simulink model "PV_panel"  (Simulink 10.0)
settings: Solver=ode45  StartTime=0.0  StopTime=0.2  RelTol=1e-3  EnableMultiTasking=on
undefined symbols (not defined in the file): sigbuilder_block
libraries: fl_lib x5, nesl_utility x5, simulink x3, ee_lib x1
settings Model: Creator=Shivananda  LastModifiedBy=bhisma
settings DataIOCC: LimitDataPoints=on  SignalLoggingSaveFormat=ModelDataLogs
settings OptimizationCC: ExpressionDepthLimit=2147483647
settings DebuggingCC: SolverPrmCheckMsg=warning  FcnCallInpInsideContextMsg=warning  StateNameClashWarn=warning
settings GRTTargetCC: GeneratePreprocessorConditionals=Disable all
settings ConfigComp: CovExternalEMLEnable=off
settings SimscapeCC: SimscapeNormalizeSystem=off

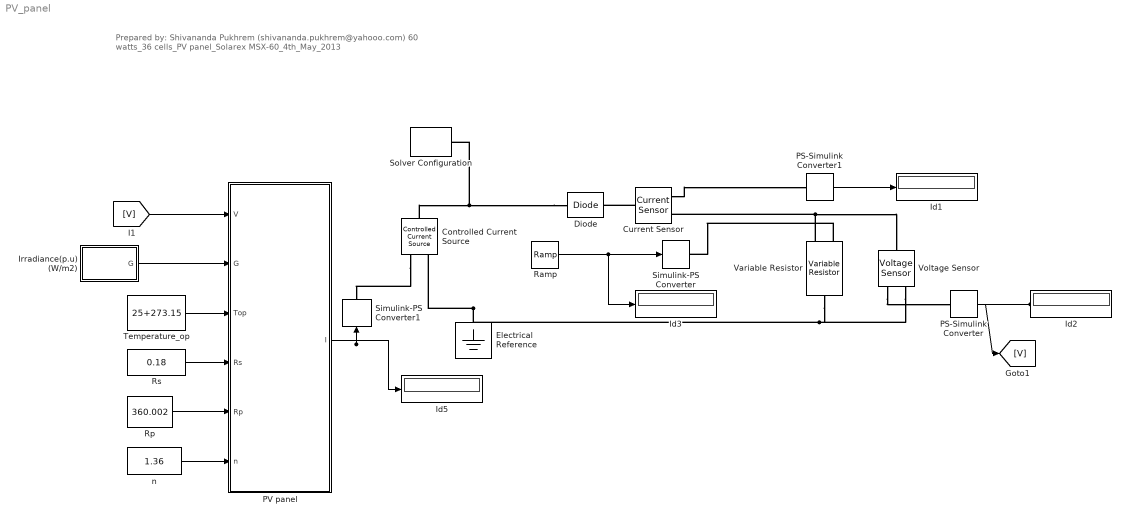
== system PV_panel ==
  note: Prepared by: Shivananda Pukhrem (shivananda.pukhrem@yahooo.com)
      |                          60 watts_36 cells_PV panel_Solarex MSX-60_4th_May_2013
  Controlled Current Source : fl_lib/Electrical/Electrical Sources/Controlled Current Source
  Current Sensor : fl_lib/Electrical/Electrical Sensors/Current Sensor
  Diode : ee_lib/Semiconductors & Converters/Diode  ModelType=ee.enum.diode.modelType.exponential  Vf=0.6 V  Ron=0.3 Ohm  Goff=1e-08 S  prmExp=1  I12="[  0.07 2.2 ] A"  V12="[  15 21 ] V"  IS=1.541765286972375e-008 A  ec=1  I1=0.07 A  V1=0.7 V  RS=0.001 Ohm  Tmeas=25 C  N_series=1  N_parallel=1  Rz=0.3 Ohm  BV=Inf V  C_param=1  CJ=0 pF  CJ0=0 pF  VJ=1 V  Mgrad=0.5  Vvec="[  0.1 10 100 ] V"  Cvec="[  3.5 1 0.4 ] pF"  FC=0.5  Q_param=ee.enum.diode.recoveryParam.off  iRM=-7.15 A  iF=4 A  didt=-750 A/us  trr_factor=3  trr=115 ns  Qrr=1500 s*uA  TT=50 ns  tau=100 ns  T_param=ee.enum.diode.temperatureParam.off  IS_T2=1.25e-7 A  I1_T2=0.245 A  V1_T2=0.5 V  Tmeas2=125 degC  EG_param=ee.enum.diode.egapParam.material_si  EG=1.11 eV  XTI_param=ee.enum.diode.xtiParam.pn  XTI=3  dBVdT=0 V/K  Tdevice=25 degC  i_specify=off  i_priority=None  i=0 A  i_nominal_specify=off  i_nominal_unit=A  i_nominal_value=1  v_specify=off  v_priority=None  v=0 V  v_nominal_specify=off  v_nominal_unit=V  v_nominal_value=1  i_capacitor_specify=off  i_capacitor_priority=None  i_capacitor=0 A  i_capacitor_nominal_specify=off  i_capacitor_nominal_unit=A  i_capacitor_nominal_value=1  v_capacitor_specify=off  v_capacitor_priority=None  v_capacitor=0 V  v_capacitor_nominal_specify=off  v_capacitor_nominal_unit=V  v_capacitor_nominal_value=1  power_dissipated_specify=off  power_dissipated_priority=None  power_dissipated=0 W  power_dissipated_nominal_specify=off  power_dissipated_nominal_unit=W  power_dissipated_nominal_value=1  thermal_network_parameterization=ee.enum.thermalNetworkTopology.cauer  Rth=[0, 10] K/W  Rth_Foster=[4, 6] K/W  thermal_mass_parameterization=ee.enum.thermalNetwork.timeconstant  thermal_mass=[0, 1] J/K  thermal_mass_Foster=[1.5, 3] J/K  thermal_time_constant=[0, 10] s  thermal_time_constant_Foster=[6, 18] s  thermal_mass_initial_temperatures=[25, 25] degC
      settings: SourceProductName=Simscape Electrical
  Electrical Reference : fl_lib/Electrical/Electrical Elements/Electrical Reference
  Id{1..3,5} (4 alike) : Display
  Irradiance(p.u) (W/m2) : Subsystem  Tag=STV Subsys  LoadFcn=sigbuilder_block('load');  StartFcn=sigbuilder_block('start');  StopFcn=sigbuilder_block('stop');  ClipboardFcn=sigbuilder_block('clipboard');  mask(Sigbuilder block){tuvar=[0:10]}
      mask help: Sigbuilder GUI
      mask init:
      | if ~strcmp(get_param(bdroot(gcbh),'SimulationStatus'),'stopped') tuvar = sigbuilder_block('maskInit'); end
      settings: CopyFcn=sigbuilder_block('copy');  DeleteFcn=sigbuilder_block('delete');  ModelCloseFcn=sigbuilder_block('modelClose');  PreSaveFcn=sigbuilder_block('preSave');  PauseFcn=sigbuilder_block('pause')  ContinueFcn=sigbuilder_block('continue')  NameChangeFcn=sigbuilder_block('namechange');  OpenFcn=sigbuilder_block('open',[518.25 6 500.25 507 ]);  CloseFcn=sigbuilder_block('close');
      mask Display: plot(0, 0, 100, 100,[2, 2, 32, 32, 2], [68, 8, 8, 68, 68],[32, 2], [38, 38], [32, 19, 2],[53, 60, 44], [32, 17, 17, 2],[16, 16, 31, 31]);txt = getActiveGroup(gcbh);text(2, 100, txt,'verticalAlignment', 'top');
  PS-Simulink Converter : nesl_utility/PS-Simulink Converter  PhysicalDomain=network_engine_domain  SubClassName=ps_output  LeftPortType=input  RightPortType=output  PseudoPeriodic=off  Frequencies=[]  Unit=1  AffineConversion=off
  PS-Simulink Converter1 : nesl_utility/PS-Simulink Converter  PhysicalDomain=network_engine_domain  SubClassName=ps_output  LeftPortType=input  RightPortType=output  PseudoPeriodic=off  Frequencies=[]  Unit=1  AffineConversion=off
  PV panel : Subsystem
  Ramp : simulink/Sources/Ramp  slope=7777  start=0  InitialOutput=0
  Rp : Constant  Value=360.002
  Rs : Constant  Value=0.18
  Simulink-PS Converter : nesl_utility/Simulink-PS Converter  PhysicalDomain=network_engine_domain  SubClassName=ps_input  LeftPortType=input  RightPortType=output  PseudoPeriodic=off  Frequencies=[]  NoiseDistribution=none  NoiseParameters=[]  Unit=1  AffineConversion=off  FilteringAndDerivatives=zero  SimscapeFilterOrder=1  InputFilterTimeConstant=.000001  UdotUserProvided=0
  Simulink-PS Converter1 : nesl_utility/Simulink-PS Converter  PhysicalDomain=network_engine_domain  SubClassName=ps_input  LeftPortType=input  RightPortType=output  PseudoPeriodic=off  Frequencies=[]  NoiseDistribution=none  NoiseParameters=[]  Unit=1  AffineConversion=off  FilteringAndDerivatives=zero  SimscapeFilterOrder=1  InputFilterTimeConstant=.000001  UdotUserProvided=0
  Solver Configuration : nesl_utility/Solver Configuration  PhysicalDomain=network_engine_domain  SubClassName=solver  LeftPortType=input  RightPortType=generic  Tones=[]  Harmonics=[]  SimulateNoise=off  Profile=off  UseLocalSampling=off  EnableSwitchedLinearOptims=on  FrequencyDomain=off  UseCCode=off  RelTol=0.001  AbsTol=1e-06  MinStep=1e-09  ToWorkspace=off  RevertToSquareIcSolve=off  NumHomotopyIterations=100  PhasorMode=off  PhasorModeNumHarmonics=1  DoDC=on  ResidualTolerance=1e-8  UseLocalSolver=on  LocalSolverChoice=NE_BACKWARD_EULER_ADVANCER  LocalSolverSampleTime=.0001  DoFixedCost=off  MaxNonlinIter=8  MaxModeIter=2  LinearAlgebra=Sparse  EquationFormulation=NE_TIME_EF  DelaysMemoryBudget=1024  AutomaticFiltering=on  FilteringTimeConstant=0.001  PartitionStorageMethod=AS_NEEDED  PartitionMemoryBudget=1024  PartitionMethod=FAST
  Temperature_op : Constant  Value=25+273.15
  Variable Resistor : fl_lib/Electrical/Electrical Elements/Variable Resistor  Rmin=0 Ohm  i_specify=off  i_priority=None  i=0 A  i_nominal_specify=off  i_nominal_unit=A  i_nominal_value=1  v_specify=off  v_priority=None  v=0 V  v_nominal_specify=off  v_nominal_unit=V  v_nominal_value=1
  Voltage Sensor : fl_lib/Electrical/Electrical Sensors/Voltage Sensor
  n : Constant  Value=1.36
  wires:
  PS-Simulink Converter/1 -> Id2/1, [V]
  PS-Simulink Converter1/1 -> Id1/1
  Ramp/1 -> Id3/1, Simulink-PS Converter/1
  PV panel/1(I) -> Simulink-PS Converter1/1, Id5/1
  Temperature_op/1 -> PV panel/3(Top)
  Rs/1 -> PV panel/4(Rs)
  Rp/1 -> PV panel/5(Rp)
  n/1 -> PV panel/6(n)
  Irradiance(p.u) (W/m2)/1(G) -> PV panel/2(G)
  [V] -> PV panel/1(V)
  connections:
  Variable Resistor/RConn1 -- Electrical Reference/LConn1 -- Controlled Current Source/RConn2 -- Voltage Sensor/RConn2
  Diode/LConn1 -- Controlled Current Source/LConn1 -- Solver Configuration/RConn1
  Variable Resistor/LConn2 -- Current Sensor/RConn2 -- Voltage Sensor/LConn1
  Voltage Sensor/RConn1 -- PS-Simulink Converter/LConn1
  Controlled Current Source/RConn1 -- Simulink-PS Converter1/RConn1
  Current Sensor/LConn1 -- Diode/RConn1
  Current Sensor/RConn1 -- PS-Simulink Converter1/LConn1
  Variable Resistor/LConn1 -- Simulink-PS Converter/RConn1

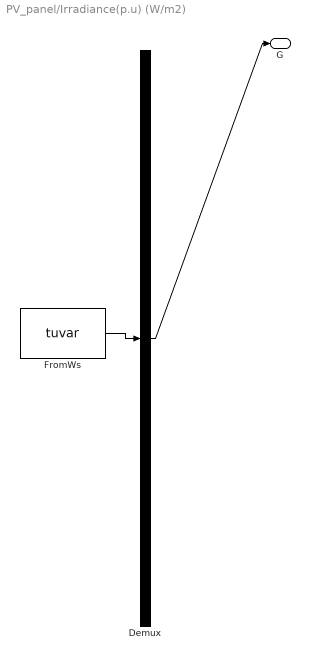
== system PV_panel/Irradiance(p.u) (W/m2) ==
  Demux : Demux  Tag=STV Demux  Outputs=1
  FromWs : FromWorkspace  Tag=STV FromWs  VariableName=tuvar  SampleTime=0  SigBuilderData=DataTag0  VnvData=DataTag1
      SigBuilderData=|
      | common.afterFinalStr = 'Extrapolate'
      | common.sampleTime = '0'
      | dataSet(1).timeRange = [0 1]
      | dataSet(1).name = 'Constant Irradiance'
      | dataSet(2).timeRange = [0 1]
      | dataSet(2).name = 'Step Irradiance'
      | dataSet(3).timeRange = [0 1]
      | dataSet(3).name = 'Trapezoidal Irradiance'
      | sbobj.Groups(1).Name = 'Constant Irradiance'
      | sbobj.Groups(1).Signals.Name = 'G'
      | sbobj.Groups(1).Signals.XData = [0 1]
      | sbobj.Groups(1).Signals.YData = [1 1]
      | sbobj.Groups(1).TimeRange = [0 1]
      | sbobj.Groups(2).Name = 'Step Irradiance'
      | sbobj.Groups(2).Signals.Name = 'G'
      | sbobj.Groups(2).Signals.XData = [0 0.5 0.5 1]
      | sbobj.Groups(2).Signals.YData = [0.6 0.6 1 1]
      | sbobj.Groups(2).TimeRange = [0 1]
      | sbobj.Groups(3).Name = 'Trapezoidal Irradiance'
      | sbobj.Groups(3).Signals.Name = 'G'
      | sbobj.Groups(3).Signals.XData = [0 0.2 0.3 0.5 0.7 0.9 1]
      | sbobj.Groups(3).Signals.YData = [0.8 0.8 0.6 0.6 1 1 0.8]
      | sbobj.Groups(3).TimeRange = [0 1]
  G : Outport  Tag=STV Outport
  wires:
  Demux/1 -> G/1
  FromWs/1 -> Demux/1

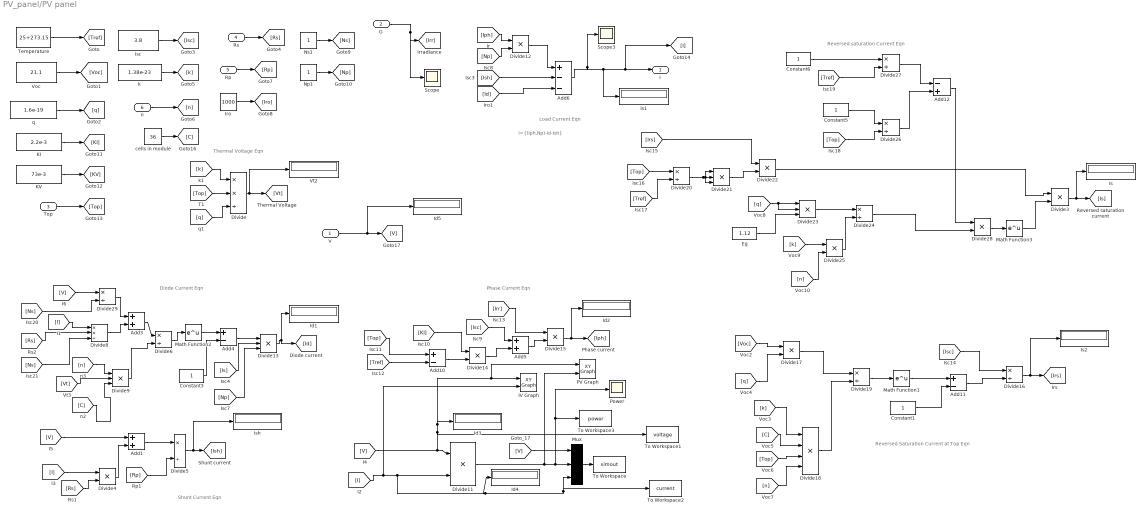
== system PV_panel/PV panel ==
  note: Diode Current Eqn
  note: Thermal Voltage Eqn
  note: Shunt Current Eqn
  note: Phase Current Eqn
  note: Load Current Eqn
  note: Reversed saturation Current Eqn
  note: Reversed Saturation Current at Top Eqn
  note: I={(Iph.Np)-Id-Ish}
  V : Inport
  G : Inport  Port=2
  Top : Inport  Port=3
  Rs : Inport  Port=4
  Rp : Inport  Port=5
  n : Inport  Port=6
  Add1 : Sum
  Add10 : Sum  Inputs=+-
  Add11 : Sum  Inputs=+-
  Add12 : Sum  Inputs=-+
  Add3 : Sum
  Add4 : Sum  Inputs=+-
  Add5 : Sum
  Add6 : Sum  Inputs=+--
  Constant{1,3,5..6} (4 alike) : Constant
  Divide : Product  Inputs=**/
  Divide{3..4,11..12,14..15,17,22,25,28} (10 alike) : Product  Inputs=**
  Divide{9,13,21,23} (4 alike) : Product  Inputs=***
  Divide{5..6,16,19..20,24,26..27,29} (9 alike) : Product  Inputs=*/
  Divide18 : Product  Inputs=****
  Divide8 : Product  Inputs=**/
  Eg : Constant  Value=1.12
  IV Graph : simulink/Sinks/XY Graph  xmin=0  xmax=23  ymin=0  ymax=4  st=-1
  Id{1..5} (5 alike) : Display
  Iro : Constant  Value=1000
  Is : Display
  Is1 : Display
  Is2 : Display
  Isc : Constant  Value=3.8
  Ish : Display
  KI : Constant  Value=2.2e-3
  KV : Constant  Value=73e-3
  Math Function1 : Math  SaturateOnIntegerOverflow=on
  Math Function2 : Math  SaturateOnIntegerOverflow=on
  Math Function3 : Math  SaturateOnIntegerOverflow=on
  Mux : Mux  Inputs=3
  Np1 : Constant
  Ns1 : Constant
  PV Graph : simulink/Sinks/XY Graph  xmin=0  xmax=23  ymin=0  ymax=61  st=-1
  Power : Scope
  Scope : Scope
  Scope3 : Scope
  Temperature : Constant  Value=25+273.15
  To Workspace : ToWorkspace  VariableName=simout  SampleTime=-1
  To Workspace1 : ToWorkspace  VariableName=voltage  SampleTime=-1
  To Workspace2 : ToWorkspace  VariableName=current  SampleTime=-1
  To Workspace3 : ToWorkspace  VariableName=power  SampleTime=-1
  Voc : Constant  Value=21.1
  Vt2 : Display
      settings: Format=long_e
  cells in module : Constant  Value=36
  k : Constant  Value=1.38e-23
  q : Constant  Value=1.6e-19
  I : Outport
  wires:
  [I] -> Divide11/2, Id4/1, Mux/3, To Workspace2/1, IV Graph/2
  Divide11/1 -> Mux/2, Power/1, To Workspace3/1, PV Graph/2
  Mux/1 -> To Workspace/1
  Temperature/1 -> [Tref]
  Voc/1 -> [Voc]
  q/1 -> [q]
  Isc/1 -> [Isc]
  k/1 -> [k]
  n/1 -> [n]
  Iro/1 -> [Iro]
  [k] -> Divide/1
  [Top] -> Divide/2
  [q] -> Divide/3
  Divide/1 -> [Vt], Vt2/1
  Divide3/1 -> Is/1, [Is]
  [Ish] -> Add6/2
  Add6/1 -> Scope3/1, Is1/1, I/1, [I]
  [I] -> Divide8/1
  [Rs] -> Divide8/2
  Divide8/1 -> Add3/2
  [n] -> Divide9/1
  [Vt] -> Divide9/2
  Divide9/1 -> Divide6/2
  Add3/1 -> Divide6/1
  Divide6/1 -> Math Function2/1
  Math Function2/1 -> Add4/1
  Constant3/1 -> Add4/2
  Add4/1 -> Divide13/1
  [Is] -> Divide13/2
  Divide13/1 -> [Id], Id1/1
  Divide4/1 -> Add1/2
  Add1/1 -> Divide5/1
  [Rp] -> Divide5/2
  Divide5/1 -> Ish/1, [Ish]
  [Rs] -> Divide4/2
  [I] -> Divide4/1
  KI/1 -> [KI]
  KV/1 -> [KV]
  [V] -> Divide11/1, To Workspace1/1, Id3/1, IV Graph/1, PV Graph/1
  [V] -> Add1/1
  [Np] -> Divide13/3
  [Iph] -> Divide12/1
  [Np] -> Divide12/2
  Divide12/1 -> Add6/1
  [Isc] -> Add5/1
  [Top] -> Add10/1
  [Tref] -> Add10/2
  Add10/1 -> Divide14/2
  [KI] -> Divide14/1
  [Irr] -> Divide15/1
  [C] -> Divide9/3
  [Isc] -> Divide16/1
  [Voc] -> Divide17/1
  [q] -> Divide17/2
  [k] -> Divide18/1
  [C] -> Divide18/2
  [Top] -> Divide18/3
  [n] -> Divide18/4
  Divide17/1 -> Divide19/1
  Divide18/1 -> Divide19/2
  Divide19/1 -> Math Function1/1
  Constant1/1 -> Add11/2
  Math Function1/1 -> Add11/1
  Add11/1 -> Divide16/2
  Divide16/1 -> [Irs], Is2/1
  [Tref] -> Divide20/2
  [Top] -> Divide20/1
  Divide20/1 -> Divide21/2, Divide21/1, Divide21/3
  Divide21/1 -> Divide22/2
  [Irs] -> Divide22/1
  [q] -> Divide23/1, Divide23/2
  Eg/1 -> Divide23/3
  Divide23/1 -> Divide24/1
  [k] -> Divide25/1
  [n] -> Divide25/2
  Divide25/1 -> Divide24/2
  Constant5/1 -> Divide26/1
  [Top] -> Divide26/2
  Constant6/1 -> Divide27/1
  [Tref] -> Divide27/2
  Divide27/1 -> Add12/1
  Divide26/1 -> Add12/2
  Add12/1 -> Divide28/1
  Divide24/1 -> Divide28/2
  Divide28/1 -> Math Function3/1
  Divide22/1 -> Divide3/1
  Math Function3/1 -> Divide3/2
  Divide29/1 -> Add3/1
  [Ns] -> Divide29/2
  [V] -> Divide29/1
  [Ns] -> Divide8/3
  Divide14/1 -> Add5/2
  Add5/1 -> Divide15/2
  Divide15/1 -> [Iph], Id2/1
  [V] -> Mux/1
  V/1 -> [V], Id5/1
  G/1 -> [Irr], Scope/1
  Top/1 -> [Top]
  cells in module/1 -> [C]
  Ns1/1 -> [Ns]
  Np1/1 -> [Np]
  [Id] -> Add6/3
  Rs/1 -> [Rs]
  Rp/1 -> [Rp]
